simulink model "EV3_motor_ident"  (Simulink 7.6)
settings: Solver=FixedStepDiscrete  StartTime=0.0  StopTime=Inf  RelTol=1e-3
InitFcn:
  | init_ident
undefined symbols (not defined in the file): Te
libraries: simulink x1, rpi_blkst x1
settings Model: Creator=jacques  LastModifiedBy=jacques  SimulationMode=external
settings OptimizationCC: OptimizeModelRefInitCode=on  LifeSpan=1
settings HardwareCC: ProdLargestAtomicInteger=Long  ProdLargestAtomicFloat=Double  ProdEndianess=LittleEndian  ProdHWDeviceType=ARM Compatible->ARM 11
settings RTWCC: SystemTargetFile=ert_rpi.tlc  TemplateMakefile=ert_rpi.tmf  PostCodeGenCommand=postGenFunc(buildInfo)  Description=RTW Embedded Coder RPI target  ProcessScript=ert_rpi_make_rtw_hook
settings CodeAppCC: IgnoreCustomStorageClasses=off
settings STFCustomTargetCC: ModelReferenceCompliant=off  CombineOutputUpdateFcns=on  ERTCustomFileBanners=on  SupportNonInlinedSFcns=off  SystemTargetFile=ert_rpi.tlc
settings ERTTargetCC: MultiwordLength=2048  ModelReferenceCompliant=off  ParMdlRefBuildCompliant=off  CompOptLevelCompliant=off  ERTFirstTimeCompliant=off  SupportContinuousTime=on  ModelStepFunctionPrototypeControlCompliant=off  CPPClassGenCompliant=off  ExtMode=on  ExtModeMexArgs='192.168.2.1'  InlinedParameterPlacement=NonHierarchical  ERTCustomFileTemplate=ert_rpi_file_process.tlc  ConvertIfToSwitch=off

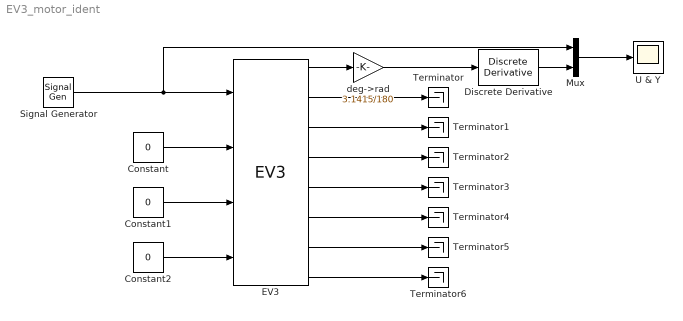
== system EV3_motor_ident ==
  Constant : Constant  Value=0  SampleTime=0.01
  Constant1 : Constant  Value=0  SampleTime=0.01
  Constant2 : Constant  Value=0  SampleTime=0.01
  Discrete Derivative : simulink/Discrete/Discrete Derivative  SystemSampleTime=-1  gainval=1.0  ICPrevScaledInput=0.0  OutMin=[]  OutMax=[]  OutDataType=fixdt(1, 16)  OutScaling=2^-10  DoSatur=off
  EV3 : rpi_blkst/EV3  SystemSampleTime=-1  rpi_mask_Ts=Te
  Mux : Mux  Inputs=2
  Signal Generator : SignalGenerator  WaveForm=square  Amplitude=50  Frequency=0.5
  Terminator{,1..6} (7 alike) : Terminator
  U & Y : Scope
      settings: YMin=-100  YMax=100  SaveName=small_motor  DataFormat=Array
  deg->rad : Gain  Gain=3.1415/180  SampleTime=Te
  wires:
  Signal Generator/1 -> EV3/1, Mux/1
  EV3/2 -> Terminator/1
  EV3/3 -> Terminator1/1
  EV3/4 -> Terminator2/1
  EV3/5 -> Terminator3/1
  EV3/6 -> Terminator4/1
  EV3/7 -> Terminator5/1
  EV3/8 -> Terminator6/1
  Constant/1 -> EV3/2
  Constant1/1 -> EV3/3
  Constant2/1 -> EV3/4
  EV3/1 -> deg->rad/1
  Mux/1 -> U & Y/1
  deg->rad/1 -> Discrete Derivative/1
  Discrete Derivative/1 -> Mux/2
